simulink model "calculate_troom_integral"  (R2016b)
settings: Solver=VariableStepAuto  StartTime=0.0  StopTime=365*24*3600  RelTol=1e-3
settings Model: Creator=drhf  LastModifiedBy=drhf

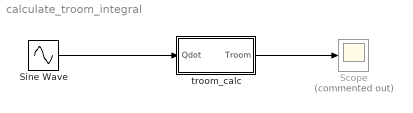
== system calculate_troom_integral ==
  Scope : Scope  Commented=on
  Sine Wave : Sin  Amplitude=1000  Frequency=2*pi/24/3600  SampleTime=0
  troom_calc : Subsystem  mask(Calculate room temperature){A=140, capa=50000, tini=20, dtroom=inf}
      mask prompts: A "Heated surface of the house in m²"; capa "Thermal capactiy per surface in J/m²/K"; tini "Initial temperature in °C"; dtroom "Max. change of room temperature in K"
      mask help:
      | One node thermal model based on energy balance.
      | The room temperature can be limited by "Max. change of room temperature" . The temperature is limited by this parameter, the result of the energy balance (Qdot_all) is the required power to maintain the limit.
      mask TypeOptions A: A/Value
      mask TypeOptions capa: capa/Value
      mask TypeOptions tini: Tini/Value | add_Tini/Bias
  wires:
  Sine Wave/1 -> troom_calc/1(Qdot)
  troom_calc/1(Troom) -> Scope/1

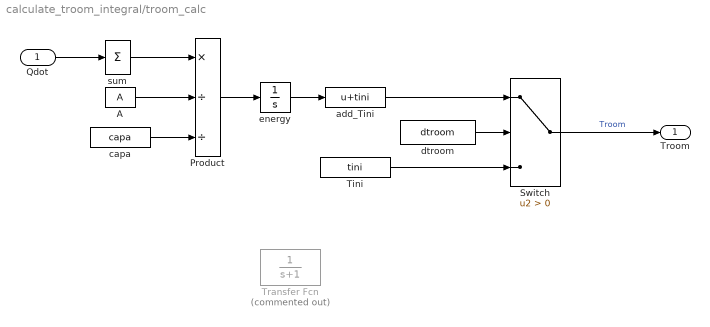
== system calculate_troom_integral/troom_calc ==
  Qdot : Inport
  A : Constant  Value=A
  Product : Product  Inputs=*//
  Switch : Switch  Criteria=u2 > Threshold
  Tini : Constant  Value=tini
  Transfer Fcn : TransferFcn  Commented=on  Denominator=[1 1]
  add_Tini : Bias  Bias=tini
  capa : Constant  Value=capa
  dtroom : Constant  Value=dtroom
  energy : Integrator  LimitOutput=on  UpperSaturationLimit=dtroom  LowerSaturationLimit=min(-dtroom, -0.01)
  sum : Sum  Inputs=1  SaturateOnIntegerOverflow=on  InputSameDT=on  OutDataTypeStr=Inherit: Same as first input
  Troom : Outport
  wires:
  sum/1 -> Product/1
  Product/1 -> energy/1
  energy/1 -> add_Tini/1
  Switch/1 -> Troom/1  "Troom"
  Qdot/1 -> sum/1
  A/1 -> Product/2
  capa/1 -> Product/3
  Tini/1 -> Switch/3
  dtroom/1 -> Switch/2
  add_Tini/1 -> Switch/1
